simulink model "PSMG2"  (R2023b)
settings: Solver=VariableStepAuto  StartTime=0.0  StopTime=0.06  RelTol=1e-3
undefined symbols (not defined in the file): J, Ke, Ld, Lq, p, Rs
libraries: mcbcontrolslib x6
settings Model: Creator=tudorn  LastModifiedBy=tudorn

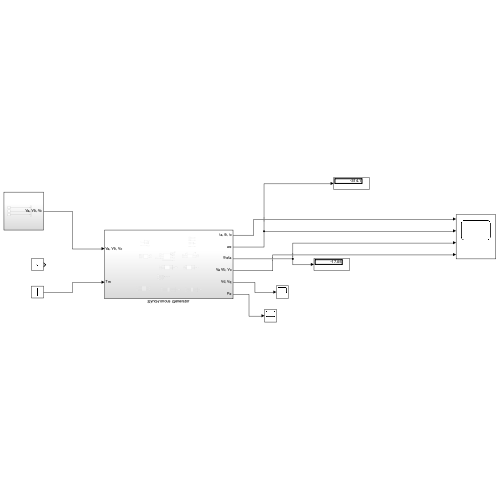
[thumbnail: Simulink's stored preview of the top-level diagram]
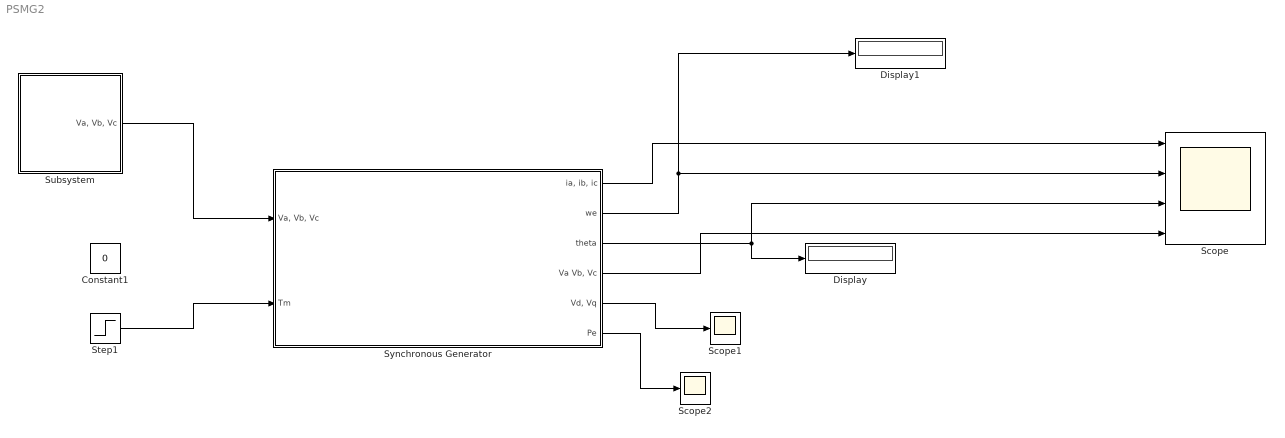
== system PSMG2 ==
  Constant1 : Constant  Value=0
  Display : Display
  Display1 : Display
  Scope : Scope  NumInputPorts=4
  Scope1 : Scope
  Scope2 : Scope
  Step1 : Step  Time=0  After=15  SampleTime=0
  Subsystem : Subsystem
  Synchronous Generator : Subsystem
  wires:
  Subsystem/1("Va, Vb, Vc") -> Synchronous Generator/1("Va, Vb, Vc")
  Step1/1 -> Synchronous Generator/2(Tm)
  Synchronous Generator/1("ia, ib, ic") -> Scope/1
  Synchronous Generator/2(we) -> Display1/1, Scope/2
  Synchronous Generator/5("Vd, Vq") -> Scope1/1
  Synchronous Generator/4("Va Vb, Vc") -> Scope/4
  Synchronous Generator/3(theta) -> Display/1, Scope/3
  Synchronous Generator/6(Pe) -> Scope2/1

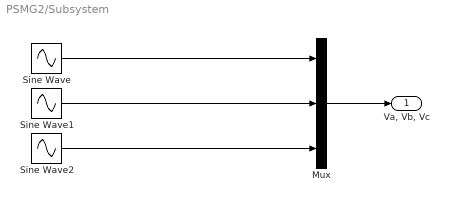
== system PSMG2/Subsystem ==
  Mux : Mux  Inputs=3
  Sine Wave : Sin  Amplitude=220  Frequency=2*pi*50  SampleTime=1e-5
  Sine Wave1 : Sin  Amplitude=220  Frequency=2*pi*50  Phase=2*pi/3  SampleTime=1e-5
  Sine Wave2 : Sin  Amplitude=220  Frequency=2*pi*50  Phase=-2*pi/3  SampleTime=1e-5
  "Va, Vb, Vc" : Outport
  wires:
  Mux/1 -> "Va, Vb, Vc"/1
  Sine Wave/1 -> Mux/1
  Sine Wave1/1 -> Mux/2
  Sine Wave2/1 -> Mux/3

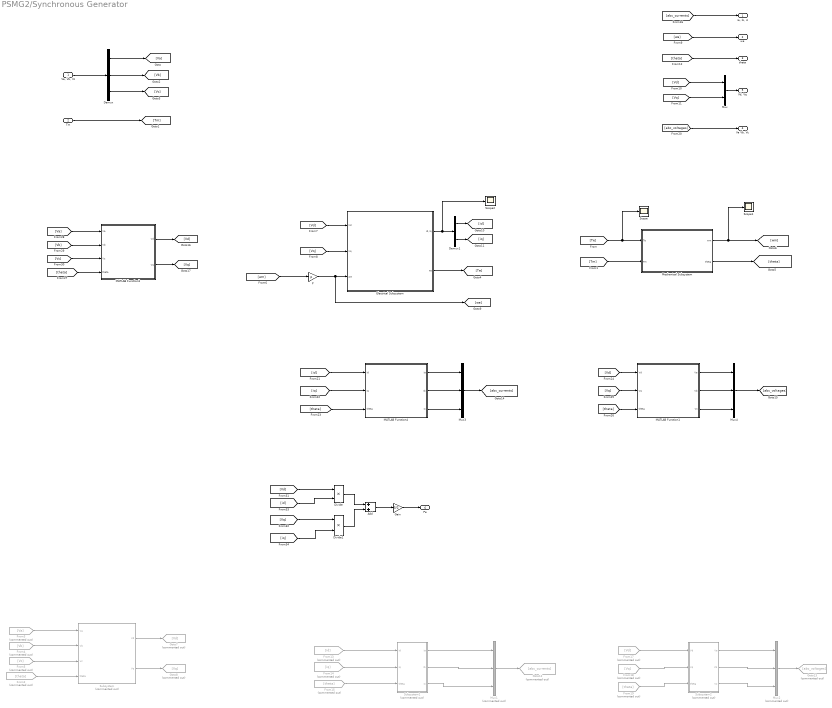
== system PSMG2/Synchronous Generator ==
  "Va, Vb, Vc" : Inport
  Tm : Inport  Port=2
  Add : Sum
  Demux : Demux  Outputs=3
  Demux1 : Demux  Outputs=2
  Divide : Product  Inputs=**
  Divide1 : Product  Inputs=**
  Electrical Subsystem : Subsystem
  From13 : From  Commented=on  GotoTag=id
  From14 : From  Commented=on  GotoTag=iq
  From15 : From  Commented=on  GotoTag=theta
  From17 : From  Commented=on  GotoTag=Vd
  From18 : From  Commented=on  GotoTag=Vq
  From19 : From  Commented=on  GotoTag=theta
  From2 : From  Commented=on  GotoTag=theta
  From3 : From  Commented=on  GotoTag=Va
  From4 : From  Commented=on  GotoTag=Vb
  From5 : From  Commented=on  GotoTag=Vc
  Gain : Gain  Gain=3/2
  Goto12 : Goto  Commented=on  GotoTag=abc_currents
  Goto13 : Goto  Commented=on  GotoTag=abc_voltages
  Goto7 : Goto  Commented=on  GotoTag=Vd
  Goto8 : Goto  Commented=on  GotoTag=Vq
  MATLAB Function1 : MATLAB Function  TreatAsAtomicUnit=on
  MATLAB Function3 : MATLAB Function  TreatAsAtomicUnit=on
  MATLAB Function4 : MATLAB Function  TreatAsAtomicUnit=on
  Mechanical Subsystem : Subsystem
  Mux : Mux  Inputs=2
  Mux1 : Mux  Commented=on  Inputs=3
  Mux2 : Mux  Commented=on  Inputs=3
  Mux3 : Mux  Inputs=3
  Mux4 : Mux  Inputs=3
  P : Gain  Gain=p
  Scope : Scope
  Scope1 : Scope
  Scope2 : Scope
  Subsystem : Subsystem  Commented=on
  Subsystem1 : Subsystem  Commented=on
  Subsystem2 : Subsystem  Commented=on
  "ia, ib, ic" : Outport
  we : Outport  Port=2
  theta : Outport  Port=3
  "Va Vb, Vc" : Outport  Port=4
  "Vd, Vq" : Outport  Port=5
  Pe : Outport  Port=6
  wires:
  "Va, Vb, Vc"/1 -> Demux/1
  Tm/1 -> [Tm]
  Demux/1 -> [Va]
  Demux/2 -> [Vb]
  Demux/3 -> [Vc]
  Electrical Subsystem/2(Te) -> [Te]
  [Te] -> Scope/1, Mechanical Subsystem/1(Te)
  [Tm] -> Mechanical Subsystem/2(Tm)
  From2/1 -> Subsystem/4(theta)
  From5/1 -> Subsystem/3(Vc)
  From4/1 -> Subsystem/2(Vb)
  From3/1 -> Subsystem/1(Va)
  Mechanical Subsystem/1(wm) -> Scope1/1, [wm]
  [wm] -> P/1
  P/1 -> [we], Electrical Subsystem/3(we)
  [Vq] -> Electrical Subsystem/2(Vq)
  [Vd] -> Electrical Subsystem/1(Vd)
  Subsystem/1(Vd) -> Goto7/1
  Subsystem/2(Vq) -> Goto8/1
  [we] -> we/1
  Mux/1 -> "Vd, Vq"/1
  [Vd] -> Mux/1
  [Vq] -> Mux/2
  [theta] -> theta/1
  Electrical Subsystem/1("id, iq") -> Scope2/1, Demux1/1
  Demux1/1 -> [id]
  Demux1/2 -> [iq]
  From13/1 -> Subsystem1/1(Id)
  Subsystem1/1(Ia) -> Mux1/1
  Subsystem1/3(Ic) -> Mux1/3
  Mux1/1 -> Goto12/1
  [abc_currents] -> "ia, ib, ic"/1
  From17/1 -> Subsystem2/1(Vd)
  From18/1 -> Subsystem2/2(Vq)
  From19/1 -> Subsystem2/3(theta)
  Subsystem2/1(Va) -> Mux2/1
  Subsystem2/2(Vb) -> Mux2/2
  Subsystem2/3(Vc) -> Mux2/3
  Mux2/1 -> Goto13/1
  [abc_voltages] -> "Va Vb, Vc"/1
  Mechanical Subsystem/2(theta) -> [theta]
  From14/1 -> Subsystem1/2(Iq)
  From15/1 -> Subsystem1/3(theta)
  Subsystem1/2(Ib) -> Mux1/2
  [iq] -> MATLAB Function4/2(Iq)
  [theta] -> MATLAB Function4/3(theta)
  [id] -> MATLAB Function4/1(Id)
  Mux3/1 -> [abc_currents]
  MATLAB Function4/2(Ib) -> Mux3/2
  MATLAB Function4/1(Ia) -> Mux3/1
  MATLAB Function4/3(Ic) -> Mux3/3
  [Vd] -> MATLAB Function1/1(Vd)
  [Vq] -> MATLAB Function1/2(Vq)
  [theta] -> MATLAB Function1/3(theta)
  Mux4/1 -> [abc_voltages]
  MATLAB Function1/1(Va) -> Mux4/1
  MATLAB Function1/2(Vb) -> Mux4/2
  MATLAB Function1/3(Vc) -> Mux4/3
  [Va] -> MATLAB Function3/1(Va)
  [Vc] -> MATLAB Function3/3(Vc)
  [theta] -> MATLAB Function3/4(theta)
  [Vb] -> MATLAB Function3/2(Vb)
  MATLAB Function3/2(Vq) -> [Vq]
  MATLAB Function3/1(Vd) -> [Vd]
  [Vq] -> Divide1/1
  [iq] -> Divide1/2
  [id] -> Divide/2
  [Vd] -> Divide/1
  Divide/1 -> Add/1
  Divide1/1 -> Add/2
  Add/1 -> Gain/1
  Gain/1 -> Pe/1

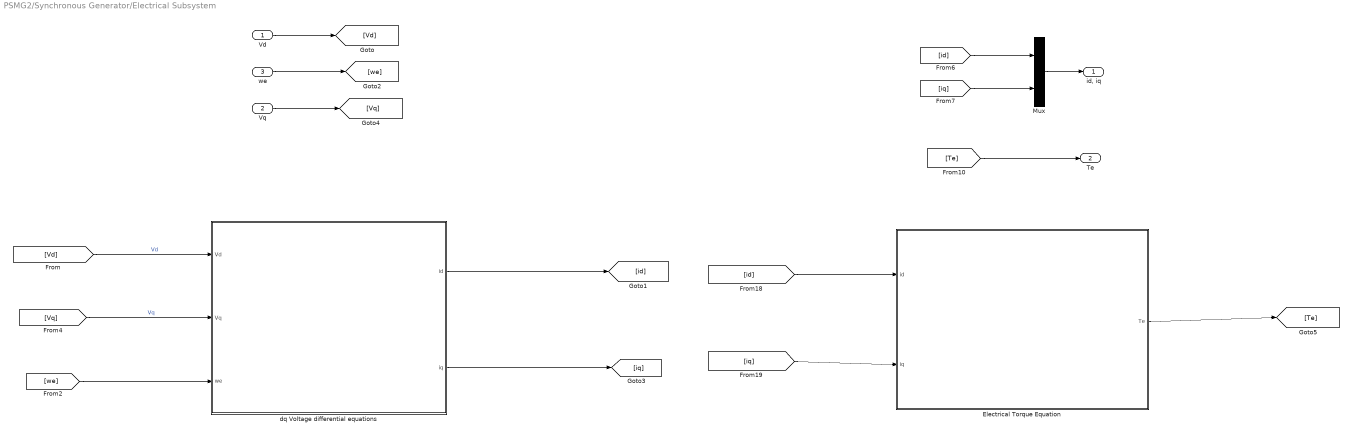
== system PSMG2/Synchronous Generator/Electrical Subsystem ==
  Vd : Inport
  Vq : Inport  Port=2
  we : Inport  Port=3
  Electrical Torque Equation : Subsystem
  Mux : Mux  Inputs=2
  dq Voltage differential equations : Subsystem
  "id, iq" : Outport
  Te : Outport  Port=2
  wires:
  Vd/1 -> [Vd]
  we/1 -> [we]
  Vq/1 -> [Vq]
  Mux/1 -> "id, iq"/1
  [id] -> Mux/1
  [iq] -> Mux/2
  [Te] -> Te/1
  [Vd] -> dq Voltage differential equations/1(Vd)  "Vd"
  [Vq] -> dq Voltage differential equations/2(Vq)  "Vq"
  dq Voltage differential equations/1(id) -> [id]
  dq Voltage differential equations/2(iq) -> [iq]
  [id] -> Electrical Torque Equation/1(id)
  [iq] -> Electrical Torque Equation/2(iq)
  Electrical Torque Equation/1(Te) -> [Te]
  [we] -> dq Voltage differential equations/3(we)

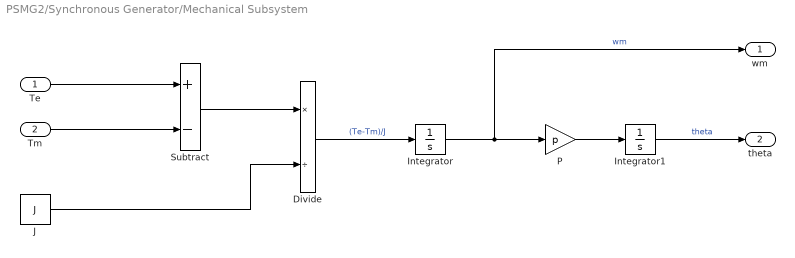
== system PSMG2/Synchronous Generator/Mechanical Subsystem ==
  Te : Inport
  Tm : Inport  Port=2
  Divide : Product  Inputs=*/
  Integrator : Integrator
  Integrator1 : Integrator
  J : Constant  Value=J
  P : Gain  Gain=p
  Subtract : Sum  Inputs=+-
  wm : Outport
  theta : Outport  Port=2
  wires:
  Tm/1 -> Subtract/2
  Te/1 -> Subtract/1
  Subtract/1 -> Divide/1
  J/1 -> Divide/2
  Divide/1 -> Integrator/1  "(Te-Tm)/J"
  Integrator/1 -> P/1, wm/1  "wm"
  Integrator1/1 -> theta/1  "theta"
  P/1 -> Integrator1/1

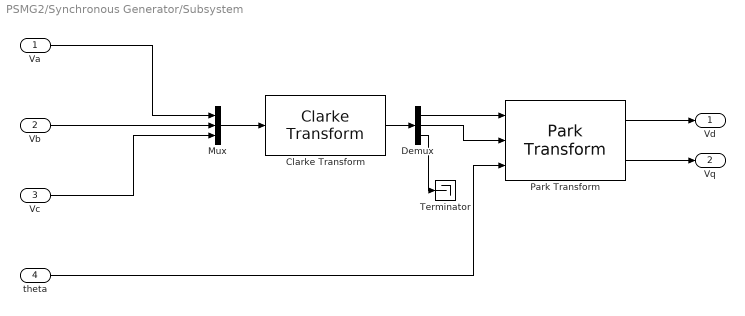
== system PSMG2/Synchronous Generator/Subsystem ==
  Va : Inport
  Vb : Inport  Port=2
  Vc : Inport  Port=3
  theta : Inport  Port=4
  Clarke Transform : mcbcontrolslib/Clarke Transform  VariantControl=Variant2  PhaseInput=Three inputs  EnPowerInv=off
      settings: LibrarySourceBlock=mcbhdllib/Controls/Math Transforms/Clarke Transform
  Demux : Demux  Outputs=3
  Mux : Mux  Inputs=3
  Park Transform : mcbcontrolslib/Park Transform  PhaseInput=Two inputs  AxisAlignment=D-axis  ThetaInput=Electrical position  AngleInput=Radians  N_points=1024
      settings: LibrarySourceBlock=mcbhdllib/Controls/Math Transforms/Park Transform
  Terminator : Terminator
  Vd : Outport
  Vq : Outport  Port=2
  wires:
  Park Transform/1 -> Vd/1
  Park Transform/2 -> Vq/1
  theta/1 -> Park Transform/3
  Mux/1 -> Clarke Transform/1
  Vc/1 -> Mux/3
  Va/1 -> Mux/1
  Vb/1 -> Mux/2
  Clarke Transform/1 -> Demux/1
  Demux/1 -> Park Transform/1
  Demux/2 -> Park Transform/2
  Demux/3 -> Terminator/1

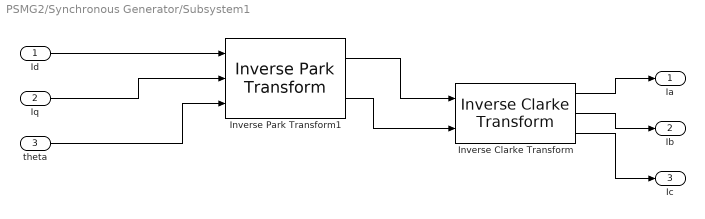
== system PSMG2/Synchronous Generator/Subsystem1 ==
  Id : Inport
  Iq : Inport  Port=2
  theta : Inport  Port=3
  Inverse Clarke Transform : mcbcontrolslib/Inverse Clarke Transform  PhaseInput=Two inputs  EnPowerInv=off
      settings: LibrarySourceBlock=mcbhdllib/Controls/Math Transforms/Inverse Clarke Transform
  Inverse Park Transform1 : mcbcontrolslib/Inverse Park Transform  PhaseInput=Two inputs  AxisAlignment=D-axis  ThetaInput=Electrical position  AngleInput=Radians  N_points=1024
      settings: LibrarySourceBlock=mcbhdllib/Controls/Math Transforms/Inverse Park Transform
  Ia : Outport
  Ib : Outport  Port=2
  Ic : Outport  Port=3
  wires:
  Id/1 -> Inverse Park Transform1/1
  Iq/1 -> Inverse Park Transform1/2
  theta/1 -> Inverse Park Transform1/3
  Inverse Park Transform1/1 -> Inverse Clarke Transform/1
  Inverse Park Transform1/2 -> Inverse Clarke Transform/2
  Inverse Clarke Transform/1 -> Ia/1
  Inverse Clarke Transform/2 -> Ib/1
  Inverse Clarke Transform/3 -> Ic/1

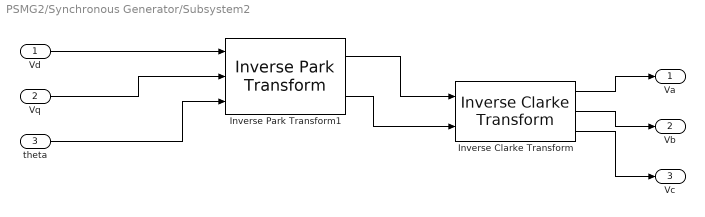
== system PSMG2/Synchronous Generator/Subsystem2 ==
  Vd : Inport
  Vq : Inport  Port=2
  theta : Inport  Port=3
  Inverse Clarke Transform : mcbcontrolslib/Inverse Clarke Transform  PhaseInput=Two inputs  EnPowerInv=off
      settings: LibrarySourceBlock=mcbhdllib/Controls/Math Transforms/Inverse Clarke Transform
  Inverse Park Transform1 : mcbcontrolslib/Inverse Park Transform  PhaseInput=Two inputs  AxisAlignment=D-axis  ThetaInput=Electrical position  AngleInput=Radians  N_points=1024
      settings: LibrarySourceBlock=mcblib/Controls/Math Transforms/Inverse Park Transform
  Va : Outport
  Vb : Outport  Port=2
  Vc : Outport  Port=3
  wires:
  Vd/1 -> Inverse Park Transform1/1
  Vq/1 -> Inverse Park Transform1/2
  theta/1 -> Inverse Park Transform1/3
  Inverse Park Transform1/1 -> Inverse Clarke Transform/1
  Inverse Park Transform1/2 -> Inverse Clarke Transform/2
  Inverse Clarke Transform/1 -> Va/1
  Inverse Clarke Transform/2 -> Vb/1
  Inverse Clarke Transform/3 -> Vc/1

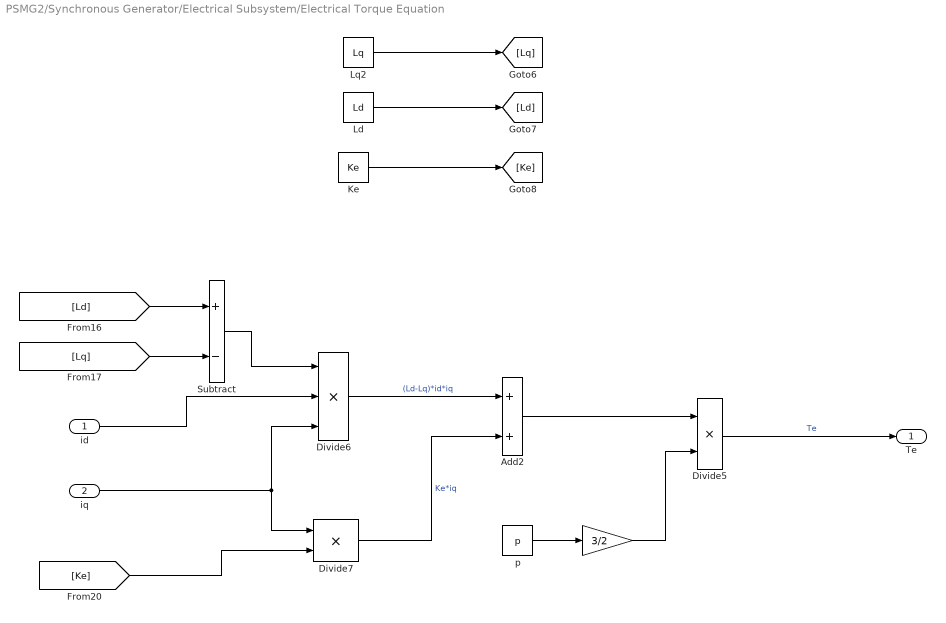
== system PSMG2/Synchronous Generator/Electrical Subsystem/Electrical Torque Equation ==
  id : Inport
  iq : Inport  Port=2
  " " : Gain  Gain=3/2
  Add2 : Sum
  Divide5 : Product  Inputs=**
  Divide6 : Product  Inputs=***
  Divide7 : Product  Inputs=**
  Ke : Constant  Value=Ke
  Ld : Constant  Value=Ld
  Lq2 : Constant  Value=Lq
  Subtract : Sum  Inputs=+-
  p : Constant  Value=p
  Te : Outport
  wires:
  id/1 -> Divide6/2
  [Ke] -> Divide7/2
  Divide5/1 -> Te/1  "Te"
  " "/1 -> Divide5/2
  iq/1 -> Divide7/1, Divide6/3
  [Ld] -> Subtract/1
  Subtract/1 -> Divide6/1
  p/1 -> " "/1
  Add2/1 -> Divide5/1
  Divide6/1 -> Add2/1  "(Ld-Lq)*id*iq"
  [Lq] -> Subtract/2
  Divide7/1 -> Add2/2  "Ke*iq"
  Ld/1 -> [Ld]
  Lq2/1 -> [Lq]
  Ke/1 -> [Ke]

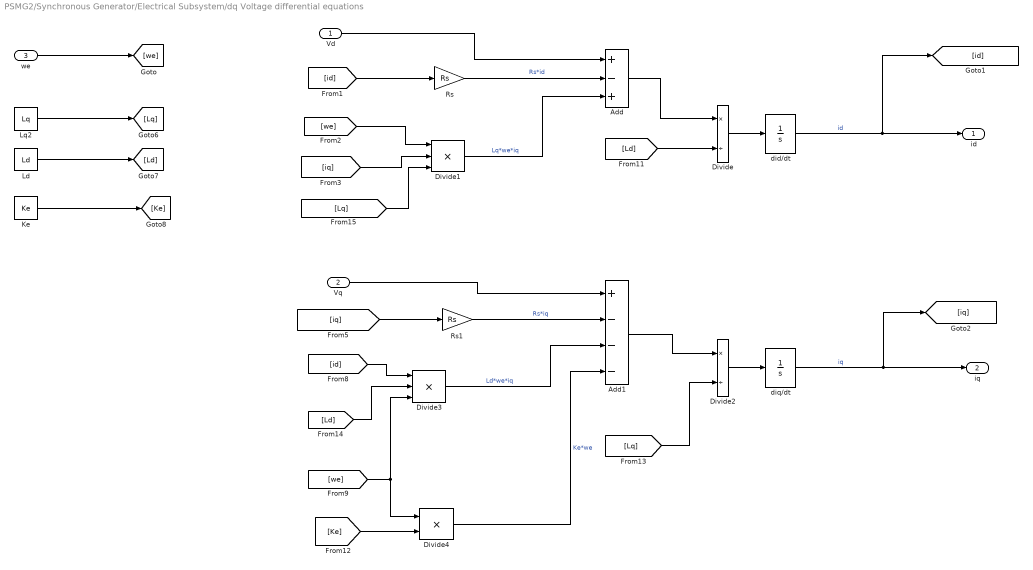
== system PSMG2/Synchronous Generator/Electrical Subsystem/dq Voltage differential equations ==
  Vd : Inport
  Vq : Inport  Port=2
  we : Inport  Port=3
  Add : Sum  Inputs=+-+
  Add1 : Sum  Inputs=+---
  Divide : Product  Inputs=*/
  Divide1 : Product  Inputs=***
  Divide2 : Product  Inputs=*/
  Divide3 : Product  Inputs=***
  Divide4 : Product  Inputs=**
  Ke : Constant  Value=Ke
  Ld : Constant  Value=Ld
  Lq2 : Constant  Value=Lq
  Rs : Gain  Gain=Rs
  Rs1 : Gain  Gain=Rs
  did/dt : Integrator
  diq/dt : Integrator
  id : Outport
  iq : Outport  Port=2
  wires:
  diq/dt/1 -> [iq], iq/1  "iq"
  Add/1 -> Divide/1
  did/dt/1 -> [id], id/1  "id"
  Rs1/1 -> Add1/2  "Rs*iq"
  [Lq] -> Divide2/2
  Vq/1 -> Add1/1
  [iq] -> Divide1/2
  [id] -> Divide3/1
  Divide1/1 -> Add/3  "Lq*we*iq"
  Add1/1 -> Divide2/1
  [iq] -> Rs1/1
  [Ld] -> Divide3/2
  Divide2/1 -> diq/dt/1
  [Lq] -> Divide1/3
  Rs/1 -> Add/2  "Rs*id"
  [we] -> Divide1/1
  Divide/1 -> did/dt/1
  [Ke] -> Divide4/2
  [we] -> Divide3/3, Divide4/1
  Divide4/1 -> Add1/4  "Ke*we"
  Divide3/1 -> Add1/3  "Ld*we*iq"
  [id] -> Rs/1
  Vd/1 -> Add/1
  [Ld] -> Divide/2
  Ld/1 -> [Ld]
  Lq2/1 -> [Lq]
  Ke/1 -> [Ke]
  we/1 -> [we]

== matlab function PSMG2/Synchronous Generator/MATLAB Function1 ==
  data: Vd input; Va output; Vq input; theta input; Vb output; Vc output
function [Va, Vb, Vc] = Inverse_ClarkePark_Voltage(Vd, Vq, theta)

    if isempty(theta)
        theta = 0;
    end

    Valpha = Vd .* cos(theta) - Vq .* sin(theta);
    Vbeta = Vd .* sin(theta) + Vq .* cos(theta);

    Va = Valpha;
    Vb = Valpha * (-1)/2 + Vbeta * sqrt(3)/2;
    Vc = Valpha * (-1)/2 - Vbeta * sqrt(3)/2;



end

== matlab function PSMG2/Synchronous Generator/MATLAB Function3 ==
  data: Va input; Vd output; Vb input; Vc input; theta input; Vq output
function [Vd, Vq] = ClarkePark(Va, Vb, Vc, theta)

    if isempty(theta)
        theta = 0;
    end
    
    Valpha = 2/3 * (Va - 0.5 * Vb - 0.5 * Vc);
    Vbeta = 2/3 * (sqrt(3)/2 * Vb - sqrt(3)/2 * Vc);

    Vd = Valpha .* cos(theta) + Vbeta .* sin(theta);
    Vq = -Valpha .* sin(theta) + Vbeta .* cos(theta);

end

== matlab function PSMG2/Synchronous Generator/MATLAB Function4 ==
  data: Id input; Ia output; Iq input; theta input; Ib output; Ic output
function [Ia, Ib, Ic] = Inverse_ClarkePark_Current(Id, Iq, theta)

    if isempty(theta)
        theta = 0;
    end

    Ialpha = Id .* cos(theta) - Iq .* sin(theta);
    Ibeta = Id .* sin(theta) + Iq .* cos(theta);

    Ia = Ialpha;
    Ib = Ialpha * (-1)/2 + Ibeta * sqrt(3)/2;
    Ic = Ialpha * (-1)/2 - Ibeta * sqrt(3)/2;


end
